simulink model "ADU_Integration_R2014a_simulation"  (R2014a)
settings: Solver=FixedStepDiscrete  StartTime=285  StopTime=300  FixedStep=0.01  RelTol=1e-3
PostLoadFcn:
  | , if any(exist('dsrtsu_mdlpostloadfcn', 'file') == [2, 3, 6]), try dsrtsu_mdlpostloadfcn('Execute', bdroot); catch fprintf('Error in PostLoadFcn (dsrtsu_mdlpostloadfcn) for model "%s":\n %s\n', bdroot, lasterr); end, end,
InitFcn:
  | load 'data/chi2_dat';
  | load 'data/Line_struct';
  | load 'data/innerLNM_1';
  | load 'data/middleLNM_2';
  | load 'data/outerLNM_1';
  | load 'data/landmarks_patac_schimmel_ccw';
  | load 'data/patac_navi_array';
  | load 'data/sensor';
  | load 'data/map_struct';
  | addpath map_src
  | Integration_Parameter;
  | load 'TestData_001';
values from neighbouring files (symbols this model uses):
  TestData_001 =     [TestData_001.mat]
undefined symbols (not defined in the file or in its folder): chi2_dat, innerLNM_1, landmarks_patac_schimmel_ccw, middleLNM_2, outerLNM_1, patac_navi_array
libraries: simulink x36, rtican x1
(part 14 of 22)

== matlab function ADU_Integration_R2014a_simulation/Path_Plan/InterSectionPathPlanningModule/PathCreater/MATLAB Function ==
  data: x_in input; y_in input; angle_in input; x_out input; y_out input; angle_out input; V_me data_store_memory; X_me data_store_memory; Y_me data_store_memory; L_me data_store_memory; W_me data_store_memory; CorLength data_store_memory; Beta data_store_memory; ratio data_store_memory; V_Ld data_store_memory; X_Ld data_store_memory; Y_Ld data_store_memory; L_Ld data_store_memory; W_Ld data_store_memory; X_CrossRl data_store_memory; Y_CrossRl data_store_memory; ArcCrossRl data_store_memory; X_CrossFr data_store_memory; Y_CrossFr data_store_memory; ArcCrossFr data_store_memory; V_Fd data_store_memory; X_Fd data_store_memory; Y_Fd data_store_memory; L_Fd data_store_memory; W_Fd data_store_memory; axlimit data_store_memory; aylimit data_store_memory; k_localmax data_store_memory; quadsinu2tbl data_store_memory; quadcosu2tbl data_store_memory; Info_Ld input; Info_Fd input; Info_Me input; xoptres output; Deltaout output; Arclengthout output; T_long output; T_lat output; PlanRes output; Delta data_store_memory; Arclength data_store_memory; Y_tar data_store_memory; KurMax output; TrigFlg input
function [xoptres,Deltaout,Arclengthout,T_long,T_lat,PlanRes,KurMax] = fcn2Inter(x_in,y_in,angle_in,x_out,y_out,angle_out,Info_Ld,Info_Fd,Info_Me,TrigFlg)
%#codegen
    global Delta W_me L_me Arclength CorLength Beta V_me Y_Ld X_Ld L_Ld W_Ld V_Ld X_Fd Y_Fd L_Fd W_Fd V_Fd X_CrossRr Y_CrossRl ArcCrossRl ArcCrossFr X_CrossFr Y_CrossFr aylimit axlimit;
    global k_localmax
    
    V_tar = 10;xoptres = 0;
    PreGlbVal(Info_Ld,Info_Fd,Info_Me,x_out,y_out,angle_out); 
    if TrigFlg > 1e-1 
        [Delta,k_localmax,Arclength] = ElementaryPathPlot( x_in,y_in,angle_in,x_out,y_out,angle_out );
        xtarFr = X_Ld -1; 
        xtarRl = X_Ld -1;
        [ ArcCrossFr,ArcCrossRl,Y_CrossFr,Y_CrossRl ] = ArcPosCalInterSection( angle_out,angle_in,x_in,y_in,x_out,y_out,0.4*Arclength,0.6*Arclength ,xtarFr,xtarRl);
        LB = [0];
        UB = [20];
        %x0 = [V_Ld];
        %xoptres = SQPCal(x0',LB',UB');
        if (4*aylimit/Arclength/Delta - V_me^2) < 1e-1
            upbound = 0;
        else
            upbound = sqrt(4*aylimit/Arclength/Delta - V_me^2);
        end
        [xoptres,hminx] = goldenSearchDirVtar(1,upbound,LB,UB);
        if hminx >= -1e-2
            V_tar = xoptres;    
            a_me = (V_tar^2 - V_me^2) /2/Arclength;
            if abs(a_me) >1e-5
                T_Cross = (V_tar - V_me)/a_me;
            else
                T_Cross = Arclength/V_me;
            end
            T_long = T_Cross ;
            T_lat =  T_Cross ;
            Deltaout = Delta;
            Arclengthout = Arclength;
            PlanRes = 1;
            KurMax = k_localmax;
        else
            xoptres = 0;Deltaout=0;Arclengthout=0;T_long=0;T_lat=0;PlanRes=0;KurMax=0;
        end
    else
        xoptres = 0;Deltaout=0;Arclengthout=0;T_long=0;T_lat=0;PlanRes=0;KurMax=0;
    end
end

function [bestStep,hminx]=goldenSearchDirVtar(lo,hi,LB,UB)
    a=lo;
    b=hi;
    error= 1e-1;
    golden=0.61803398;
    goldenn = 0;
    alpha=a + (1-golden) * (b-a);
    beta=a + golden * (b-a);    
    [f_alpha,hminx_alpha]=Pfunc( alpha,LB,UB);
    [f_beta,hminx_beta]=Pfunc( beta,LB,UB);

    while(abs(b-a)>error)
        goldenn = goldenn + 1;
    %     a1=a;  b1=b;
        if alpha>beta
    %         a=a1;b=b1;
            alpha=a + (1-golden) * (b-a);
            beta=a + golden * (b-a);
            [f_alpha,hminx_alpha]=Pfunc( alpha,LB,UB);
            [f_beta,hminx_beta]=Pfunc( beta,LB,UB);       
        end  
        if f_alpha<=f_beta
            b=beta;
            beta=alpha;
            f_beta=f_alpha;
            alpha=a + (b-beta);
            [f_alpha,hminx_alpha]=Pfunc( alpha,LB,UB);
    %         a1=a;  b1=b;
        else
            a = alpha;
            alpha = beta;
            f_alpha = f_beta;
            beta = b - (alpha-a);
            [f_beta,hminx_beta] = Pfunc( beta,LB,UB);
    %         a1=a;  b1=b;
        end
    end
    goldenn 
    bestStep = (a + b)/2;
    hminx = (hminx_beta + hminx_alpha)/2;
%     if Pfunc(a,LB,UB)<Pfunc(b,LB,UB)
%         bestStep=a;
%     else
%         bestStep=b;
%     end
end

function xoptim = SQPCal(x0,LB,UB)

    global ratio
    ratio = 1e3;
    ic = 0
    N1flg = 0;
    limit1 = 0;    limit2 = 0;
    lolimit = 0;      hilimit = 0;
    dk = [1]'; Lamda = ones(6,1);  x1 = x0;Bk=eye(1);xoptim = x0;
    while (1)
        if N1flg == 0
            [CostG,ConG,Costx,Hx]=GradientCal(x0,LB,UB);
            N1flg =1;
            Alpha = 1;
        else
            for i = 1:1
                if abs(dk(i)) < 1e-4
                    limit1 = 0;
                    limit2 = 1e4;                
                else
                    limit1 = ((LB(i) - x1(i))./dk(i));
                    limit2 = ((UB(i) - x1(i))./dk(i));
                end
                lolimit = min([limit1(i),limit2(i)]);
                hilimit = max([limit1(i),limit2(i)]);
            end
            Lo = max([lolimit,0]);
            Hi = min(hilimit);
            if (Hi <0)||(Hi < Lo)
                break;
            end
            Alpha=goldenSearch(x1,dk,Lo,Hi,LB,UB);
            if Alpha == 0
                break;
            end
            x1temp = x1;
            x1 = x1 + Alpha * dk;
            sk=x1-x1temp; 
            initial_CostG = LxGradientCal(x1temp,Lamda,LB,UB);
            CostG = LxGradientCal(x1,Lamda,LB,UB);
            yk = CostG-initial_CostG; 

            if  yk'*sk>0
                Bk=Bk+(sk*sk')/(yk'*sk)-(Bk*yk*yk'*Bk)/(yk'*Bk*yk);  
            else 
                %Bk=Bk;
            end   
            [CostG,ConG,Costx,Hx] = GradientCal(x1,LB,UB);
        end
        y1 = ones(6,1);
        w1 = ones(6,1);
        dx1 = 1;

        [dk,Lamda] = qpfunc( Bk,CostG,ConG',-Hx,dx1,y1,w1 );  
        if (norm(dk,2)<1e-3)||(Alpha < 1e-4)
            xoptim = x1;
            break;
        end
    end
end

function [CostG,ConG,Costx,Hx]= GradientCal(Xin,LB,UB)

    value1Cost=0;
    value2Cost=0;
    value1Con=[0 0 0 0 0 0];
    value2Con=[0 0 0 0 0 0];
    dx=1e-1;
    Xin_x=Xin+ dx;
    value1Cost = (  CostFun(Xin_x) - CostFun(Xin) ) / dx;    
    ConFuncXinVal = ConFunc(Xin,LB,UB);
    value1Con(1,:) = (  ConFunc(Xin_x,LB,UB) - ConFuncXinVal ) / dx;    
    Xin_x=Xin-dx;
    value2Cost = (  CostFun(Xin_x) - CostFun(Xin) ) / (-dx);   
    value2Con(1,:) = (  ConFunc(Xin_x,LB,UB) - ConFuncXinVal ) / (-dx);    
    CostG = (value2Cost + value1Cost)/2;
    ConG = (value2Con + value1Con)/2;
    Costx = CostFun(Xin);
    Hx = ConFuncXinVal;
end

function bestStep=goldenSearch(x0,direction,lo,hi,LB,UB)
    a=lo;
    b=hi;
    error=1e-3;
    golden=0.61803398;

    alpha=a + (1-golden) * (b-a);
    beta=a + golden * (b-a);
    [f_alpha,hminx_alpha]=Pfunc( x0 + alpha * direction,LB,UB);
    [f_beta,hminx_beta]=Pfunc( x0 + beta * direction,LB,UB);

    while(abs(b-a)>error)
    %     a1=a;  b1=b;
        if alpha>beta
    %         a=a1;b=b1;
            alpha=a + (1-golden) * (b-a);
            beta=a + golden * (b-a);
            [f_alpha,hminx_alpha]=Pfunc( x0 + alpha * direction,LB,UB);
            [f_beta,hminx_beta]=Pfunc( x0 + beta * direction,LB,UB);       
        end  
        if f_alpha<=f_beta
            b=beta;
            beta=alpha;
            f_beta=f_alpha;
            alpha=a + (b-beta);
            [f_alpha,hminx_alpha]=Pfunc( x0 + alpha*direction,LB,UB);
    %         a1=a;  b1=b;
        else
            a = alpha;
            alpha = beta;
            f_alpha = f_beta;
            beta = b - (alpha-a);
            [f_beta,hminx_beta] = Pfunc( x0 + beta * direction,LB,UB);
    %         a1=a;  b1=b;
        end

    end

%     if Pfunc(x0 + a * direction,LB,UB)<Pfunc(x0 + b * direction,LB,UB)
%         bestStep=a;
%     else
%         bestStep=b;
%     end
end

function [dk,dkLamda] = qpfunc( H,c,A,b,x1,y1,w1 )
%UNTITLED2 Summary of this function goes here
%   Detailed explanation goes here
Delta = 0.1;
P = 0.9;
E = ones(length(y1),1);
m = length(b);
k = 0;
    while(1)
        k = k + 1
        if k == 245
            k = k;
        end
        Y = diag(y1);
        W = diag(w1);
        Rho = b - A*x1 + w1;
        Sigma = c + H*x1 -A'*y1;
        Gamma = y1'*w1;
        Mu = Delta * Gamma / m;
        newMatricL = [-H A';A inv(Y)*W];
        newMatricR = [c + H*x1 - A'*y1;b-A*x1 + Mu*inv(Y)*E];
        dxy = inv(newMatricL)*newMatricR;
        dx = dxy(1:length(x1));
        dy = dxy((length(x1)+1):(length(dxy)));
        dw = inv(Y)*(Mu*E - Y*W*E - W*dy);
        LamdaTemp1 = [-dy./y1,-dw./w1];
        Lamda = min([1, P*pinv(max([-dy./y1;-dw./w1]))]);
        %if ((norm(Rho,1)>1e-2)|(norm(Sigma,1)>1e-2))
        if (norm(Gamma,1)<1e-3)&(norm(Rho,1)<1e-3)&(norm(Sigma,1)<1e-3)
            dk = x1;
            dkLamda = y1;
            break;
        else
            if Lamda < 1e-4
                dk = x1;
                dkLamda = y1;
                break;                
            else
                x1 = x1 + Lamda*dx;
                y1 = y1 + Lamda*dy;
                w1 = w1 + Lamda*dw;
            end
        end
    end
end

function dLxVal= LxGradientCal(Xin,Lamda,LB,UB)
    value1LxVal = 0;
    value2LxVal = 0;
    dx=1e-1;
    Xin_x=Xin+ dx;    
    ConFuncValue = ConFunc(Xin_x,LB,UB);
    value1LxVal = (CostFun(Xin_x) - CostFun(Xin)- Lamda' *  ConFunc(Xin_x,LB,UB) + Lamda' *  ConFuncValue)/dx;
    Xin_x=Xin-dx;
    value2LxVal = -(CostFun(Xin_x) - CostFun(Xin)- Lamda' *  ConFunc(Xin_x,LB,UB) + Lamda' *  ConFuncValue)/dx;
    dLxVal = (value1LxVal + value2LxVal)/2;
    dLxVal = dLxVal';    
end

% function  Pval = Pfunc2(Xin,LB,UB)
%     global ratio 
%     C = ConFunc(Xin,LB,UB)
%     hminx= min([0,min(-C)]);
%     Pval = InterSectionCostFunc(Xin) + ratio* norm(hminx,1);
% end

function  [Pval,hminx] = Pfunc(Xin,LB,UB)
    global ratio 
    C = ConFunc(Xin,LB,UB)
    hminx= min([0,min(-C)]);
    Pval = InterSectionCostFunc(Xin) + ratio* norm(hminx,1);
end

function Fcost= CostFun(Xin)
    Fcost = InterSectionCostFunc(Xin);
end

function ConVal= ConFunc(Xin,LB,UB)
    C = [0 0 0 0 0 0];
    [C(1:4),Ceq] = InterSectionNon( Xin);
    LengthC = 4;
    LengthLB = length(LB);
    C((LengthC+1):(LengthC+LengthLB))= Xin - UB;
    C((LengthC+LengthLB+1):(LengthC+LengthLB+LengthLB))= LB - Xin;
%     C=-C;
    ConVal = C';
end

function [ ArcFr,ArcRl,ypositionFr,ypositionRl ] = ArcPosCalInterSection( angle_out,angle_in,x_in,y_in,x_out,y_out,x0,x1 ,xtarFr,xtarRl)

    xpositionFr = 0;ypositionFr = 0;xpositionRl = 0;ypositionRl = 0; 
    xpositionFrtemp = 0;ypositionFrtemp = 0;xpositionRltemp = 0;ypositionRltemp = 0; 
    temp1 = x0;
    temp2 = x1;
    [xpositionFrtemp,ypositionFrtemp,xpositionRltemp,ypositionRltemp] = InterSectionPosCal( x0,angle_out,angle_in,x_in,y_in,x_out,y_out,1 );
    funx0 = xpositionFrtemp - xtarFr;
    [xpositionFrtemp,ypositionFrtemp,xpositionRltemp,ypositionRltemp] = InterSectionPosCal( x1,angle_out,angle_in,x_in,y_in,x_out,y_out,1 );
    funx1 = xpositionFrtemp - xtarFr;
    x2 = x1-funx1*(x1-x0)/(funx1-funx0);
    Sectn = 0;
    while (abs(x1-x0)>=1.0e-1) && (Sectn<=20) 
        x0=x1;                                       
        x1=x2; 
        [xpositionFrtemp,ypositionFrtemp,xpositionRltemp,ypositionRltemp] = InterSectionPosCal( x0,angle_out,angle_in,x_in,y_in,x_out,y_out,2 );
        funx0 = xpositionFrtemp - xtarFr;
        [xpositionFrtemp,ypositionFrtemp,xpositionRltemp,ypositionRltemp] = InterSectionPosCal( x1,angle_out,angle_in,x_in,y_in,x_out,y_out,2 );
        funx1 = xpositionFrtemp - xtarFr;
        x2 = x1-funx1*(x1-x0)/(funx1-funx0);
        Sectn=Sectn+1;
    end
    Sectn 
    ArcFr = x2;
    ypositionFr = ypositionFrtemp;   
    
%     x0 = temp1;
    x0 = x2;
    x1 = temp2;
    
    [xpositionFrtemp,ypositionFrtemp,xpositionRltemp,ypositionRltemp] = InterSectionPosCal( x0,angle_out,angle_in,x_in,y_in,x_out,y_out,3 );
    funx0 = xpositionRltemp - xtarRl;
    [xpositionFrtemp,ypositionFrtemp,xpositionRltemp,ypositionRltemp] = InterSectionPosCal( x1,angle_out,angle_in,x_in,y_in,x_out,y_out,3 );
    funx1 = xpositionRltemp - xtarRl;
    x2 = x1-funx1*(x1-x0)/(funx1-funx0);
    Sectn = 0;
    while (abs(x1-x0)>=1.0e-1) && (Sectn<=20)      
        x0=x1;                                      
        x1=x2;                                       
        %x2=x1-fun(x1)*(x1-x0)/(fun(x1)-fun(x0));            
        [xpositionFrtemp,ypositionFrtemp,xpositionRltemp,ypositionRltemp] = InterSectionPosCal( x0,angle_out,angle_in,x_in,y_in,x_out,y_out,3 );
        funx0 = xpositionRltemp - xtarRl;
        [xpositionFrtemp,ypositionFrtemp,xpositionRltemp,ypositionRltemp] = InterSectionPosCal( x1,angle_out,angle_in,x_in,y_in,x_out,y_out,3 );
        funx1 = xpositionRltemp - xtarRl;
        x2 = x1-funx1*(x1-x0)/(funx1-funx0);
        Sectn=Sectn+1;
    end 
    Sectn
    ArcRl = x2;
    ypositionRl = ypositionRltemp;
end

function [xpositionFr,ypositionFr,xpositionRl,ypositionRl] = InterSectionPosCal( Arc,angle_out,angle_in,x_in,y_in,x_out,y_out,Num )
%UNTITLED3 Summary of this function goes here
%   Detailed explanation goes here
%   Num == 1 Calculate All
%   Num == 0 Calculate None
%   Num == 2 Calculate Fr only
%   Num == 3 Calculate Rl only
    global Delta Arclength
    global L_me W_me
    xpositionFr = 0;
    ypositionFr = 0;
    xpositionRl = 0;
    ypositionRl = 0;
    switch Num
        case 0,
            FrCal = 0;
            RlCal = 0;
        case 1,
            FrCal = 1;
            RlCal = 1;
        case 2,
            FrCal = 1;
            RlCal = 0;
        case 3,
            FrCal = 0;
            RlCal = 1;  
    end    
    if FrCal || RlCal   
         [xposition,yposition,Theta] = ElementaryPosCal( Arc,Delta,Arclength,angle_out,angle_in,x_in,y_in,x_out,y_out );     
        if FrCal
            xpositionFr = xposition + L_me * cos(Theta) + W_me * sin(Theta) / 2;
            ypositionFr = yposition + L_me * sin(Theta) - W_me * cos(Theta) / 2;
        else
            xpositionFr = 0;ypositionFr = 0;
        end        
        if RlCal
            xpositionRl = xposition - W_me * sin(Theta) / 2;
            ypositionRl = yposition + W_me * cos(Theta) / 2;
        else
            xpositionRl = 0;ypositionRl = 0;
        end
    else
        xpositionFr = 0;ypositionFr = 0;xpositionRl = 0;ypositionRl = 0;
    end
end

function [Delta,k_localmax,Arclength] = ElementaryPathPlot( x_in,y_in,angle_in,x_out,y_out,angle_out )
    Beta = (angle_out - angle_in)/2;
    r = sqrt((x_in-x_out)^2+(y_in-y_out)^2);   
    SignBeta = sign(Beta);
    Beta = abs(Beta);
    ulimit = sqrt(Beta);
    D_BetaVal = sin(Beta)*quadsinu2(ulimit)+cos(Beta)*quadcosu2(ulimit);
    %Droot = fzero(@(x) sin(x)*quadsinu2(x)+cos(x)*quadcosu2(x), pi);
    Delta = 8*SignBeta*D_BetaVal^2/r^2;
    %longth of the trajectary     
    Arclength = 2*sqrt(2*abs(Beta/Delta*SignBeta));
    k_localmax = Delta * Arclength/2;    
end

function [xposition,yposition,Theta] = ElementaryPosCal( Arc,Delta,Arclength,angle_out,angle_in,x_in,y_in,x_out,y_out )
%UNTITLED Summary of this function goes here
%   Detailed explanation goes here   
    Beta = (angle_out - angle_in)/2;
    theta_rot = angle_in;
    x_outRot = (x_out - x_in)*cos(theta_rot) + (y_out - y_in)*sin(theta_rot);
    y_outRot = (y_out - y_in)*cos(theta_rot) - (x_out - x_in)*sin(theta_rot);    
    if Beta == 0
        SignBeta = 1;
    else
        SignBeta = sign(Beta);
    end
    if Arc < Arclength/2    
        ulimit = Arc * sqrt(abs(Delta)/2);
        Theta = Delta * (Arc)^2/2;
        xpositionTemp = sqrt(2/abs(Delta))*quadcosu2(ulimit);
        ypositionTemp = sqrt(2/abs(Delta))*quadsinu2(ulimit) * SignBeta;
    else
        ulimit = (Arclength - Arc) * sqrt(abs(Delta)/2); 
        %Theta = 2*Beta*SignBeta - Delta * (Arclength - Arc)^2/2; 
        xpositionMirrTemp = sqrt(2/abs(Delta))*quadcosu2(ulimit);
        ypositionMirrTemp = sqrt(2/abs(Delta))*quadsinu2(ulimit) * SignBeta;
        %mirror line Ax+By+C=0
        x_mirr = (x_outRot)/2;
        y_mirr = (y_outRot)/2;
        angle_mirr = pi/2 + atan((y_outRot)/(x_outRot));
        A = tan(angle_mirr);
        B = -1;
        C = y_mirr - A * x_mirr;      
        %two points are symmetrical to the Ax+By+C we just defined
        xpositionTemp = xpositionMirrTemp - 2*A*(A*xpositionMirrTemp+B*ypositionMirrTemp+C)/(A^2+B^2);
        ypositionTemp = ypositionMirrTemp - 2*B*(A*xpositionMirrTemp+B*ypositionMirrTemp+C)/(A^2+B^2);
        Theta = 2*abs(Beta)*SignBeta - Delta * (Arclength - Arc)^2/2;          
    end
    theta_rot = - angle_in;   
    xposition = xpositionTemp*cos(theta_rot) + ypositionTemp*sin(theta_rot);
    yposition = ypositionTemp*cos(theta_rot) - xpositionTemp*sin(theta_rot) ;  
    xposition = xposition + x_in;
    yposition = yposition + y_in;
    Theta = Theta + angle_in;    
end

function quadcosu2val = quadcosu2( ulimit )
    %UNTITLED4 Summary of this function goes here
    %   Detailed explanation goes here
    % this function is used to calculate the integral of cos(x^2),which is used
    % to calculate x position
    global quadcosu2tbl
    index = fix(ulimit/0.0005) + 1;
    quadcosu2val = quadcosu2tbl(index);
end

function quadsinu2val = quadsinu2( ulimit )
%UNTITLED4 Summary of this function goes here
%   Detailed explanation goes here
% this function is used to calculate the integral of sin(x^2),which is used
% to calculate y position
    global quadsinu2tbl 
    index = fix(ulimit/0.0005) + 1;
    quadsinu2val = quadsinu2tbl(index);
end

function cost = InterSectionCostFunc( Xin )
    %UNTITLED2 Summary of this function goes here
    %   Detailed explanation goes here
    cost = - Xin;

end

function [ C,Ceq ] = InterSectionNon( Xin )
    %UNTITLED Summary of this function goes here
    %   Detailed explanation goes here
    %   Non linear constraints of intersection
    global Delta W_me L_me Arclength CorLength Beta V_me Y_Ld X_Ld L_Ld W_Ld V_Ld X_Fd Y_Fd L_Fd W_Fd V_Fd X_CrossRr Y_CrossRl ArcCrossRl ArcCrossFr X_CrossFr Y_CrossFr aylimit axlimit;
    global X_me Y_me X_tar Y_tar
    Tc = [0 0];
    C=[0 0 0 0];
    MSS = [0 0];
    CRootFrLd = [0 0 0];
    CRootRrFd = [0 0 0];
    r = sqrt(2)*CorLength;
    V_tar = Xin;
    a_me = (V_tar^2 - V_me^2) /2/Arclength;
    V_CrossRr = sqrt(V_me^2 + 2*a_me*ArcCrossRl);
    if abs(a_me) >1e-5
        T_CrossRr = (V_CrossRr-V_me)/a_me;
        T_Cross = (V_tar - V_me)/a_me;
    else
        T_CrossRr = ArcCrossRl/V_me;
        T_Cross = Arclength/V_me;
    end
    V_CrossFr = sqrt(V_me^2 + 2*a_me*ArcCrossFr);
    if abs(a_me) >1e-5
        T_CrossFr = (V_CrossFr-V_me)/a_me;
    else
        T_CrossFr = Y_CrossFr/V_Ld;
    end
    Tc(1) = T_CrossFr;
    Tc(2) = T_CrossRr;    
    T_lat = T_Cross;
    T_long = T_lat;
    T_adj = 0;
    
    MSS(1) = MSSFdJudgment( V_tar,V_me,V_Fd,T_lat,Tc(1),T_lat,T_adj );
    MSS(2) = MSSLdJudgment( V_tar,V_me,V_Ld,T_lat,Tc(2),T_lat,T_adj );    
    Y_meTemp = - Arclength + Y_tar;    
    MSSFdlimitC = Y_Fd - Y_meTemp + L_Fd + MSS(1);
    MSSLdlimitC = MSS(2) + Y_meTemp + L_me - Y_Ld;
        Xin
        MSS
    C(1) = MSSFdlimitC;
    C(2) = MSSLdlimitC;
    % local vehicle position is calculated approximately, using Y = Ax + B, by
    % solving the local position - Fd/Ld position, we can judge whether the two
    % vehicle will collide in the process 
    %TnearFr = fzero(@(t) (Y_Ld + V_Ld * T_CrossFr - L_Ld + V_Ld * t) - (CorLength + L_me - Y_CrossFr) / (Arclength - ArcCossFr) * (V_CrossFr*t + a_me * t^2 /2) - Y_CrossFr,0);
%     CRootFrLd(3) = Y_Ld + V_Ld * T_CrossFr - L_Ld - Y_CrossFr;
%     CRootFrLd(2) = V_Ld - (CorLength + L_me - Y_CrossFr) / (Arclength - ArcCrossFr) * V_CrossFr;
%     CRootFrLd(1) = (CorLength + L_me - Y_CrossFr) / (Arclength - ArcCrossFr) * (a_me / 2 );
%     %TnearRr = fzero(@(t) (Y_Fd + V_Fd * T_CrossRr + V_Fd * t) - (CorLength - Y_CrossRl) / (Arclength - ArcCossRr) * (V_CrossRr*t + a_me * t^2 /2) - Y_CrossRl,0);
%     CRootRrFd(3) = Y_Fd + V_Fd * T_CrossRr - Y_CrossRl;
%     CRootRrFd(2) = V_Fd - (CorLength - Y_CrossRl) / (Arclength - ArcCrossRl) * V_CrossRr;
%     CRootRrFd(1) = (CorLength - Y_CrossRl) / (Arclength - ArcCrossRl) * (a_me /2);
%     % Judge whether the time to collide lies within T_cross, if not, the path
%     % will be considered as a safe path
%     if (CRootFrLd(2)^2-4*CRootFrLd(3)*CRootFrLd(1)) >= 0
%         RootFrLdtemp = roots(CRootFrLd);
%         RootFrLd = real(RootFrLdtemp);
%         if CRootFrLd(1) ==0
%             RootFrLd(2) = RootFrLd(1);
%         end
%         if(RootFrLd(2)>= 0)
%             C(1) = -(RootFrLd(2) + T_CrossFr) + T_Cross;
%         elseif(RootFrLd(1) >= 0)
%             C(1) = -(RootFrLd(1) + T_CrossFr) + T_Cross;        
%         else
%             C(1) = -1;
%         end
%     else
%         C(1) = -1;    
%     end
%     if (CRootRrFd(2)^2-4*CRootRrFd(3)*CRootRrFd(1)) >= 0
%         RootRrFdtemp = roots(CRootRrFd);
%         RootRrFd = real(RootRrFdtemp);
%         if CRootRrFd(1) ==0
%             RootRrFd(2) = RootRrFd(1);
%         end
%         if(RootRrFd(2)>= 0)
%             C(2) = -(RootRrFd(2) + T_CrossRr) + T_Cross;
%         elseif(RootRrFd(1) >= 0)
%             C(2) = -(RootRrFd(1) + T_CrossRr) + T_Cross;        
%         else
%             C(2) = -1;
%         end
%     else
%         C(2) = -1; 
%     end
    % ay is calculated approximately using the half Arclength position, where
    % the corning radius is the smallest
%     C(3) = V_CrossFr^2 * Delta * Arclength/2 - aylimit;
    C(3) = (V_tar^2 + V_me^2)/2 * Delta * Arclength/2 - aylimit;
    C(4) = abs(a_me) - axlimit;
    Ceq = [];

end

function MSS = MSSFdJudgment( V_tar,V_me,V_obj,T_long,Tc,T_lat,T_adj )
%UNTITLED5 Summary of this function goes here
%   Detailed explanation goes here
    
    if abs(V_me-V_tar)<1e-5
    
        if V_me>V_obj
            MSS = (-V_me+V_obj)*(Tc+T_adj);
        else
            MSS = (-V_me+V_obj)*(T_adj+T_lat);
        end
        
    else

        T_max = (V_obj - V_me)/(V_tar - V_me)*T_long;
        MSSTemp1 = 0;
        MSSTemp2 = 0;

        if Tc < T_long
            if (V_obj >= V_tar)&&(V_tar >V_me)
                MSS = MSSCalculate( V_tar,V_me,V_obj,T_long,T_lat,0 ,T_adj);
            elseif (V_obj >= V_me)&&(V_me > V_tar)
                MSS = MSSCalculate( V_tar,V_me,V_obj,T_long,T_lat,0 ,T_adj);
            elseif (V_me >= V_obj)&&(V_obj >= V_tar)
                if Tc > T_max
                    MSS = MSSCalculate( V_tar,V_me,V_obj,T_long,T_lat,0 ,T_adj);
                else
                    MSSTemp1 = MSSCalculate( V_tar,V_me,V_obj,T_long,T_lat,0 ,T_adj);  
                    MSSTemp2 = MSSCalculate( V_tar,V_me,V_obj,T_long,Tc,0 ,T_adj);
                    MSS = max(MSSTemp1,MSSTemp2);           
                end

            elseif (V_obj <= V_tar)&&(V_tar < V_me)
                MSS = MSSCalculate( V_tar,V_me,V_obj,T_long,Tc,0 ,T_adj);

            elseif (V_obj <= V_me)&&(V_me < V_tar)
                MSS = MSSCalculate( V_tar,V_me,V_obj,T_long,Tc,0 ,T_adj);

            elseif (V_me <= V_obj)&&(V_obj <= V_tar)
                if Tc > T_max
                    MSS = MSSCalculate( V_tar,V_me,V_obj,T_long,Tc,0 ,T_adj);
                else 
                    MSS = MSSCalculate( V_tar,V_me,V_obj,T_long,T_max,0 ,T_adj);
                end            
            else
                %Nothing
                MSS = 255;
            end    
        else
            % Tc > T_long
            if  V_tar > V_obj
                MSS = MSSCalculate( V_tar,V_me,V_obj,T_long,Tc,0 ,T_adj);
            else
                MSS = MSSCalculate( V_tar,V_me,V_obj,T_long,T_lat,0 ,T_adj);
            end  
        end
    end
    
end

function MSS = MSSFoJudgment( V_tar,V_me,V_obj,T_long,Tc,T_lat,T_adj )
%UNTITLED5 Summary of this function goes here
%   Detailed explanation goes here

    if abs(V_me-V_tar)<1e-5

        if V_me>V_obj
            MSS = 0;
        else
            MSS = (-V_me+V_obj)*(T_adj+Tc);
        end

    else
        T_max = (V_obj - V_me)/(V_tar - V_me)*T_long;
        MSSTemp1 = 0;
        MSSTemp2 = 0;
        if Tc < T_long
            if (V_obj >= V_tar)&&(V_tar >V_me)
                MSS = MSSCalculate( V_tar,V_me,V_obj,T_long,Tc,0 ,T_adj);
            elseif (V_obj >= V_me)&&(V_me >V_tar)
                MSS = MSSCalculate( V_tar,V_me,V_obj,T_long,Tc,0 ,T_adj);
            elseif (V_me >= V_obj)&&(V_obj >= V_tar)
                if Tc > 2*T_max
                    MSS = MSSCalculate( V_tar,V_me,V_obj,T_long,Tc,0 ,T_adj);
                else
                    MSS = 0;           
                end

            elseif (V_obj <= V_tar)&&(V_tar < V_me)
                %MSS = MSSCalculate( V_tar,V_me,V_obj,T_long,0,0 );
                MSS = 0;

            elseif (V_obj <= V_me)&&(V_me < V_tar)
                %MSS = MSSCalculate( V_tar,V_me,V_obj,T_long,0,0 );
                MSS = 0;
            elseif (V_me <= V_obj)&&(V_obj <= V_tar)
                if Tc > T_max
                    MSS = MSSCalculate( V_tar,V_me,V_obj,T_long,T_max,0 ,T_adj);
                else 
                    MSS = MSSCalculate( V_tar,V_me,V_obj,T_long,Tc,0 ,T_adj);
                end            
            else
                %Nothing
                MSS = 255;
            end    
        else
            % Tc > T_long
            if (V_obj >= V_tar)&&(V_tar >V_me)
                MSS = MSSCalculate( V_tar,V_me,V_obj,T_long,Tc,0 ,T_adj);

            elseif (V_obj >= V_me)&&(V_me >V_tar)
                MSS = MSSCalculate( V_tar,V_me,V_obj,T_long,Tc,0 ,T_adj);

            elseif (V_me >= V_obj)&&(V_obj >= V_tar)
                MSSTemp1 = 0;  
                MSSTemp2 = MSSCalculate( V_tar,V_me,V_obj,T_long,Tc,0 ,T_adj);
                MSS = max(MSSTemp1,MSSTemp2);  

            elseif (V_obj <= V_tar)&&(V_tar < V_me)
                MSS = 0;

            elseif (V_obj <= V_me)&&(V_me < V_tar)
                MSS = 0;

            elseif (V_me <= V_obj)&&(V_obj <= V_tar)
                MSS = MSSCalculate( V_tar,V_me,V_obj,T_long,T_max,0 ,T_adj);           
            else
                %Nothing
                MSS = 255;
            end  
        end
    end
end

function MSS = MSSLdJudgment( V_tar,V_me,V_obj,T_long,Tc,T_lat,T_adj )
%UNTITLED5 Summary of this function goes here
%   Detailed explanation goes here

    if abs(V_me-V_tar)<1e-5
    
        if V_me>V_obj
            MSS = (V_me-V_obj)*(T_lat+T_adj);
        else
            MSS = (V_me-V_obj)*(T_adj+Tc);
        end

    else
        T_max = (V_obj - V_me)/(V_tar - V_me)*T_long;
        MSSTemp1 = 0;
        MSSTemp2 = 0;

        if Tc < T_long
            if (V_obj >= V_tar)&&(V_tar >V_me)
                MSS = MSSCalculate( V_tar,V_me,V_obj,T_long,Tc,1 ,T_adj);

            elseif (V_obj >= V_me)&&(V_me >V_tar)
                MSS = MSSCalculate( V_tar,V_me,V_obj,T_long,Tc,1 ,T_adj);

            elseif (V_me >= V_obj)&&(V_obj >= V_tar)
                if Tc > T_max
                    MSS = MSSCalculate( V_tar,V_me,V_obj,T_long,Tc,1 ,T_adj);
                else
                    % Tc < T_max
                    MSS = MSSCalculate( V_tar,V_me,V_obj,T_long,T_max,1 ,T_adj);            
                end

            elseif (V_obj <= V_tar)&&(V_tar < V_me)
                MSS = MSSCalculate( V_tar,V_me,V_obj,T_long,T_lat,1 ,T_adj);

            elseif (V_obj <= V_me)&&(V_me < V_tar)
                MSS = MSSCalculate( V_tar,V_me,V_obj,T_long,T_lat,1 ,T_adj);

            elseif (V_me <= V_obj)&&(V_obj <= V_tar)
                MSSTemp1 = MSSCalculate( V_tar,V_me,V_obj,T_long,T_lat,1 ,T_adj);  
                MSSTemp2 = MSSCalculate( V_tar,V_me,V_obj,T_long,Tc,1 ,T_adj);
                MSS = max(MSSTemp1,MSSTemp2);

            else
                %Nothing
                MSS = 255;
            end    
        else
            % Tc > T_long
            if V_obj > V_tar
                MSS = MSSCalculate( V_tar,V_me,V_obj,T_long,Tc,1 );

            else
                MSS = MSSCalculate( V_tar,V_me,V_obj,T_long,T_lat,1 );

            end    
        end
    end
end

function MSS = MSSLoJudgment( V_tar,V_me,V_obj,T_long,Tc,T_lat,T_adj )
%UNTITLED5 Summary of this function goes here
%   Detailed explanation goes here
    if abs(V_me-V_tar)<1e-5
        if V_me>V_obj
            MSS = (V_me-V_obj)*(Tc+T_adj);
        else
            MSS = 0;
        end
    else
        T_max = (V_obj - V_me)/(V_tar - V_me)*T_long;
        MSSTemp1 = 0;
        MSSTemp2 = 0;

        if Tc < T_long
            if (V_obj >= V_tar)&&(V_tar >V_me)
                %MSS = MSSCalculate( V_tar,V_me,V_obj,T_long,0,1 );
                MSS = 0;
            elseif (V_obj >= V_me)&&(V_me >V_tar)
                %MSS = MSSCalculate( V_tar,V_me,V_obj,T_long,0,1 );
                MSS = 0;
            elseif (V_me >= V_obj)&&(V_obj >= V_tar)
                if Tc > T_max
                    MSS = MSSCalculate( V_tar,V_me,V_obj,T_long,T_max,1 ,T_adj);
                else
                    % Tc < T_max
                    MSS = MSSCalculate( V_tar,V_me,V_obj,T_long,Tc,1 ,T_adj);            
                end

            elseif (V_obj <= V_tar)&&(V_tar < V_me)
                MSS = MSSCalculate( V_tar,V_me,V_obj,T_long,Tc,1 ,T_adj);

            elseif (V_obj <= V_me)&&(V_me < V_tar)
                MSS = MSSCalculate( V_tar,V_me,V_obj,T_long,Tc,1 ,T_adj);

            elseif (V_me <= V_obj)&&(V_obj <= V_tar)
                if Tc < 2*T_max
                    %MSS = MSSCalculate( V_tar,V_me,V_obj,T_long,0,1 );              
                    MSS = 0;
                else 
                    MSS = MSSCalculate( V_tar,V_me,V_obj,T_long,Tc,1 ,T_adj);
                end            
            else
                %Nothing
                MSS = 255;
            end    
        else
            % Tc > T_long
            if (V_obj >= V_tar)&&(V_tar >V_me)
                %MSS = MSSCalculate( V_tar,V_me,V_obj,T_long,0,1 );
                MSS = 0;
            elseif (V_obj >= V_me)&&(V_me >V_tar)
                %MSS = MSSCalculate( V_tar,V_me,V_obj,T_long,0,1 );
                MSS = 0;
            elseif (V_me >= V_obj)&&(V_obj >= V_tar)
                MSS = MSSCalculate( V_tar,V_me,V_obj,T_long,T_max,1 ,T_adj);

            elseif (V_obj <= V_tar)&&(V_tar < V_me)
                MSS = MSSCalculate( V_tar,V_me,V_obj,T_long,Tc,1 ,T_adj);

            elseif (V_obj <= V_me)&&(V_me < V_tar)
                MSS = MSSCalculate( V_tar,V_me,V_obj,T_long,Tc,1 ,T_adj);

            elseif (V_me <= V_obj)&&(V_obj <= V_tar)
                MSSTemp1 = 0;  
                MSSTemp2 = MSSCalculate( V_tar,V_me,V_obj,T_long,Tc,1 ,T_adj);
                MSS = max(MSSTemp1,MSSTemp2);           
            else
                %Nothing
                MSS = 255;
            end  
        end
    end
end

function MSS = MSSCalculate( V_tar,V_me,V_obj,T_long,Time2Cal,ObjDirection ,T_adj)
%UNTITLED3 Summary of this function goes here
%   Detailed explanation goes here

%Time2Cal is the time to be calculated
%V_tar is the target of mergeing vehicle
%V_obj is the obstacle object of mergeing vehicle
%ObjDirection is the direction of object
%T_long is the time when longitual vel adjust ends

    if Time2Cal < T_long
        MSS = (V_tar-V_me)/2/T_long*Time2Cal^2-(V_obj-V_me)*Time2Cal;
    else
        MSS = (V_tar-V_me)/2*T_long - (V_obj - V_me)*T_long - (V_obj - V_tar)*Time2Cal;
    end

    if ObjDirection == 1
        %obj is Leading vehicle 
    else
        %obj is Following vehicle
        MSS = (-1)*MSS;
    end
end

function PreGlbVal(Info_Ld,Info_Fd,Info_Me,x_out,y_out,angle_out)
    global Delta W_me L_me Arclength CorLength Beta V_me Y_Ld X_Ld L_Ld W_Ld V_Ld X_Fd Y_Fd L_Fd W_Fd V_Fd X_CrossRr Y_CrossRl ArcCrossRl ArcCrossFr X_CrossFr Y_CrossFr aylimit axlimit;
    global quadsinu2tbl quadcosu2tbl Y_tar ratio
    %Config doublecheck of the safe judgement when driving through intersection
    %Config plot the process or not
    %Config check the accuracy of y postion estimate
    %cor start point at intersection which is also the Radius of the intersection
    persistent InitFlg
    if isempty(InitFlg)
        InitFlg = 0;
    end
    CorLength = 20;
    ratio = 1e3;
    %the 1/2 direction changed in the intersection   
%     x_out,y_out,angle_out;
    if abs(Info_Ld(3))>100
        %Invalid Leading vehicle
        X_Ld = x_out;
        Y_Ld = y_out + 100;
        V_Ld = 30;
        L_Ld = 2.5;
        W_Ld = 1.5; 
    else
        X_Ld = Info_Ld(1);
        Y_Ld = Info_Ld(2);
        V_Ld = Info_Ld(3);
        L_Ld = Info_Ld(4);
        W_Ld = Info_Ld(5); 
    end
    if abs(Info_Fd(3))>100
        %Invalid Leading vehicle
        X_Fd = x_out;
        Y_Fd = y_out - 100;
        V_Fd = 0;
        L_Fd = 2.5;
        W_Fd = 1.5; 
    else 
        X_Fd = Info_Fd(1);
        Y_Fd = Info_Fd(2);
        V_Fd = Info_Fd(3);
        L_Fd = Info_Fd(4);
        W_Fd = Info_Fd(5); 
    end

    X_me = Info_Me(1);
    Y_me = Info_Me(2);
    V_me = Info_Me(3);
    L_me = Info_Me(4);
    W_me = Info_Me(5);   
    Y_tar = 20;
    aylimit = 3;
    axlimit = 2;
    
    ArcCrossFr = 0;
    ArcCrossRl = 0;
    Y_CrossFr = 0;
    Y_CrossRl = 0;
    if InitFlg < 1e-1
